simulink model "three_ringnetwork_with_control"  (R2016a)
settings: Solver=VariableStepAuto  StartTime=0.0  StopTime=0.2  RelTol=1e-3
undefined symbols (not defined in the file): vc0d
libraries: simulink x18, powerlib_meascontrol x3
(part 1 of 3)
settings Model: Creator=r-manohar  LastModifiedBy=r-manohar

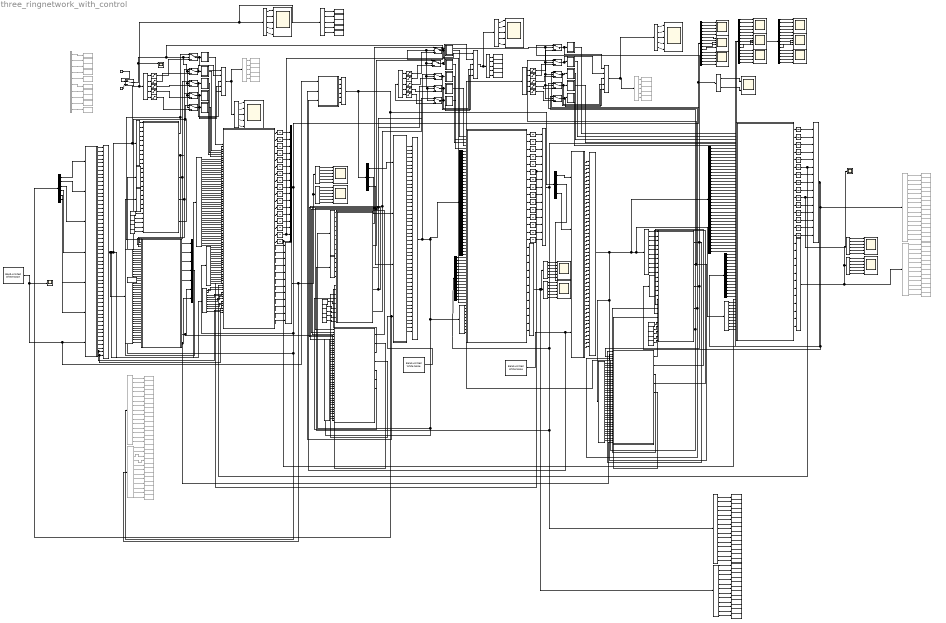
== system three_ringnetwork_with_control ==
  note: ab
  note: bc
  note: ca
  " Switch" : ManualSwitch
  Band-Limited White Noise : simulink/Sources/Band-Limited White Noise  Cov=[0.07]  Ts=0.01  seed=[234321]
  Band-Limited White Noise1 : simulink/Sources/Band-Limited White Noise  Cov=[0.07]  Ts=0.01  seed=[23341]
  Band-Limited White Noise2 : simulink/Sources/Band-Limited White Noise  Cov=[0.07]  Ts=0.01  seed=[2314441]
  Bus Creator1 : BusCreator  Inputs=17
  Bus Creator10 : BusCreator  Inputs=7
  Bus Creator11 : BusCreator  Inputs=6
  Bus Creator12 : BusCreator  Inputs=5
  Bus Creator13 : BusCreator  Inputs=5
  Bus Creator14 : BusCreator  Inputs=5
  Bus Creator2 : BusCreator  Inputs=56
  Bus Creator3 : BusCreator  Inputs=15
  Bus Creator4 : BusCreator  Inputs=12
  Bus Creator5 : BusCreator  Inputs=15
  Bus Creator6 : BusCreator  Inputs=12
  Bus Creator7 : BusCreator  Inputs=12
  Bus Creator8 : BusCreator  Inputs=50
  Bus Creator9 : BusCreator  Inputs=50
  Bus Selector1 : BusSelector  OutputSignals=E0,E1,E2,E3,E4,R1t0,R1t1,R1t2,R1t3,R1t4,R2t0,R2t1,R2t2,R2t3,R2t4,C0,C1,C2,C3,C4,L0,L1,L2,L3,L4,Lt0,Lt1,Lt2,Lt3,Lt4,il0d,il1d,il2d,il3d,il4d
  Bus Selector10 : BusSelector  OutputSignals=U0,U1,U2,U3,U4
  Bus Selector11 : BusSelector  OutputSignals=H,H0,H1,H2,H3,H4
  Bus Selector12 : BusSelector  OutputSignals=He0,He1,He2,He3,He4,He
  Bus Selector13 : BusSelector  OutputSignals=H,H0,H1,H2,H3,H4
  Bus Selector14 : BusSelector  OutputSignals=signal1,signal2,signal3,signal4,signal5,signal6,signal7,signal8,signal9,signal10,signal11,signal12,signal13,signal14,signal15,signal16,signal17
  Bus Selector{15..16,22..23,26,31,43..44} (8 alike) : BusSelector  OutputSignals=signal1,signal2,signal3,signal4,signal5
  Bus Selector17 : BusSelector  OutputSignals=He0,He1,He2,He3,He4,He
  Bus Selector18 : BusSelector  Commented=on  OutputSignals=signal1,signal2,signal3,signal4,signal5
  Bus Selector19 : BusSelector  OutputSignals=H,H0,H1,H2,H3,H4
  Bus Selector2 : BusSelector  OutputSignals=E0,E1,E2,E3,E4,R1t0,R1t1,R1t2,R1t3,R1t4,R2t0,R2t1,R2t2,R2t3,R2t4,C0,C1,C2,C3,C4,L0,L1,L2,L3,L4,Lt0,Lt1,Lt2,Lt3,Lt4,il0d,il1d,il2d,il3d,il4d,Rab,Lab,Rac,Lac
  Bus Selector20 : BusSelector  OutputSignals=vc0ss,vc1ss,vc2ss,vc3ss,vc4ss,ilt0ss,ilt1ss,ilt2ss,ilt3ss,ilt4ss
  Bus Selector21 : BusSelector  OutputSignals=E0,E1,E2,E3,E4,il0d,il1d,il2d,il3d,il4d
  Bus Selector24 : BusSelector  OutputSignals=R1t0,R1t1,R1t2,R1t3,R1t4,R2t0,R2t1,R2t2,R2t3,R2t4,il0d,il1d,il2d,il3d,il4d,C0,C1,C2,C3,C4,Lt0,Lt1,Lt2,Lt3,Lt4,vc0ss,vc1ss,vc2ss,vc3ss,vc4ss,ilt0ss,ilt1ss,ilt2ss,ilt3ss,ilt4ss,Lab,Lac,Rab,Rac,iabss,iacss
  Bus Selector25 : BusSelector  OutputSignals=E0,E1,E2,E3,E4,il0d,il1d,il2d,il3d,il4d
  Bus Selector{3,6..7,27,32,47} (6 alike) : BusSelector  OutputSignals=signal1,signal2,signal3,signal4,signal5,signal6,signal7,signal8,signal9,signal10,signal11,signal12,signal13,signal14,signal15
  Bus Selector28 : BusSelector  OutputSignals=R1t0,R1t1,R1t2,R1t3,R1t4,R2t0,R2t1,R2t2,R2t3,R2t4,il0d,il1d,il2d,il3d,il4d,C0,C1,C2,C3,C4,Lt0,Lt1,Lt2,Lt3,Lt4,vc0ss,vc1ss,vc2ss,vc3ss,vc4ss,ilt0ss,ilt1ss,ilt2ss,ilt3ss,ilt4ss
  Bus Selector29 : BusSelector  OutputSignals=R1t0,R1t1,R1t2,R1t3,R1t4,R2t0,R2t1,R2t2,R2t3,R2t4,il0d,il1d,il2d,il3d,il4d,C0,C1,C2,C3,C4,Lt0,Lt1,Lt2,Lt3,Lt4,vc0ss,vc1ss,vc2ss,vc3ss,vc4ss,ilt0ss,ilt1ss,ilt2ss,ilt3ss,ilt4ss
  Bus Selector30 : BusSelector  OutputSignals=E0,E1,E2,E3,E4,il0d,il1d,il2d,il3d,il4d
  Bus Selector33 : BusSelector  OutputSignals=Eb0,Rab,Ea0
  Bus Selector34 : BusSelector  OutputSignals=Ec0,Rac,Ea1
  Bus Selector35 : BusSelector  OutputSignals=Rab,Rac,Ea0,Ea1,Eb0,Ec0
  Bus Selector36 : BusSelector  OutputSignals=U0,U1,U2,U3,U4
  Bus Selector37 : BusSelector  OutputSignals=U0,U1,U2,U3,U4
  Bus Selector38 : BusSelector  Commented=on  OutputSignals=signal1,signal2,signal3,signal4,signal5,signal6,signal7,signal8,signal9,signal10,signal11,signal12,signal13,signal14,signal15
  Bus Selector39 : BusSelector  OutputSignals=signal16,signal17
  Bus Selector4 : BusSelector  OutputSignals=vc0ss,vc1ss,vc2ss,vc3ss,vc4ss,ilt0ss,ilt1ss,ilt2ss,ilt3ss,ilt4ss
  Bus Selector40 : BusSelector  Commented=on  OutputSignals=He0,He1,He2,He3,He4,He,H,H0,H1,H2,H3,H4
  Bus Selector41 : BusSelector  Commented=on  OutputSignals=E0,E1,E2,E3,E4,R2t0,R2t1,R2t2,R2t3,R2t4
  Bus Selector42 : BusSelector  OutputSignals=E0,E1,E2,E3,E4
  Bus Selector45 : BusSelector  OutputSignals=E0,E1,E2,E3,E4
  Bus Selector46 : BusSelector  Commented=on  OutputSignals=signal1,signal2,signal3,signal4,signal5
  Bus Selector48 : BusSelector  OutputSignals=He0,He1,He2,He3,He4,He,H,H0,H1,H2,H3,H4
  Bus Selector49 : BusSelector  Commented=on  OutputSignals=signal1,signal2,signal3,signal4,signal5,signal6,signal7,signal8,signal9,signal10,signal11,signal12,signal13,signal14,signal15
  Bus Selector5 : BusSelector  OutputSignals=E0,E1,E2,E3,E4,R1t0,R1t1,R1t2,R1t3,R1t4,R2t0,R2t1,R2t2,R2t3,R2t4,C0,C1,C2,C3,C4,L0,L1,L2,L3,L4,Lt0,Lt1,Lt2,Lt3,Lt4,il0d,il1d,il2d,il3d,il4d
  Bus Selector50 : BusSelector  Commented=on  OutputSignals=He0,He1,He2,He3,He4,He,H,H0,H1,H2,H3,H4
  Bus Selector8 : BusSelector  OutputSignals=vc0ss,vc1ss,vc2ss,vc3ss,vc4ss,ilt0ss,ilt1ss,ilt2ss,ilt3ss,ilt4ss
  Bus Selector9 : BusSelector  OutputSignals=He0,He1,He2,He3,He4,He
  Init : MATLAB Function  TreatAsAtomicUnit=on
  Init1 : MATLAB Function  TreatAsAtomicUnit=on
  Init2 : MATLAB Function  TreatAsAtomicUnit=on
  MATLAB Function : MATLAB Function  TreatAsAtomicUnit=on
  PWM0 : Subsystem
  PWM1 : Subsystem
  PWM10 : Subsystem
  PWM11 : Subsystem
  PWM12 : Subsystem
  PWM13 : Subsystem
  PWM14 : Subsystem
  PWM2 : Subsystem
  PWM3 : Subsystem
  PWM4 : Subsystem
  PWM5 : Subsystem
  PWM6 : Subsystem
  PWM7 : Subsystem
  PWM8 : Subsystem
  PWM9 : Subsystem
  Ralpha : Constant  Value=20
  Ralpha1 : Constant  Value=20
  Ralpha2 : Constant  Value=20
  Rbeta : Constant  Value=20
  Rbeta1 : Constant  Value=20
  Rbeta2 : Constant  Value=20
  Rdelta : Constant  Value=20
  Rdelta1 : Constant  Value=20
  Rdelta2 : Constant  Value=20
  Reta : Constant  Value=20
  Reta1 : Constant  Value=20
  Reta2 : Constant  Value=20
  Rgamma : Constant  Value=20
  Rgamma1 : Constant  Value=20
  Rgamma2 : Constant  Value=20
  Saturation{,1..14} (15 alike) : Saturate  UpperLimit=1  LowerLimit=0
  Scope : Scope
  Scope1 : Scope  NumInputPorts=2
  Scope4 : Scope  NumInputPorts=2
  Switch{,1..14} (15 alike) : Switch  Criteria=u2 > Threshold  Threshold=0.5
  cont : Subsystem
  cont1 : Subsystem
  cont2 : Subsystem
  controll : Constant
  h : Scope  NumInputPorts=6
  h1 : Scope  NumInputPorts=6
  h2 : Scope  NumInputPorts=6
  he : Scope  NumInputPorts=6
  he0_file1 : ToFile  Commented=on  Filename=E0.mat  MatrixName=E0_tr
  he0_file10 : ToFile  Filename=E0.mat  MatrixName=E0_tr
  he0_file11 : ToFile  Filename=h4.mat  MatrixName=h4_tr
  he0_file12 : ToFile  Commented=on  Filename=h4.mat  MatrixName=h4_tr
  he0_file13 : ToFile  Commented=on  Filename=he0.mat  MatrixName=he0_tr
  he0_file14 : ToFile  Commented=on  Filename=h3.mat  MatrixName=h3_tr
  he0_file15 : ToFile  Commented=on  Filename=h0.mat  MatrixName=h0_tr
  he0_file2 : ToFile  Commented=on  Filename=R2t0.mat  MatrixName=R2t0_tr
  he0_file3 : ToFile  Commented=on  Filename=he0.mat  MatrixName=he0_tr
  he0_file4 : ToFile  Commented=on  Filename=h3.mat  MatrixName=h3_tr
  he0_file5 : ToFile  Commented=on  Filename=h0.mat  MatrixName=h0_tr
  he0_file6 : ToFile  Commented=on  Filename=h4.mat  MatrixName=h4_tr
  he0_file7 : ToFile  Filename=he0.mat  MatrixName=he0_tr
  he0_file8 : ToFile  Filename=h3.mat  MatrixName=h3_tr
  he0_file9 : ToFile  Filename=h0.mat  MatrixName=h0_tr
  he1 : Scope  NumInputPorts=6
  he1_file1 : ToFile  Filename=he1.mat  MatrixName=he1_tr
  he1_file10 : ToFile  Commented=on  Filename=E2.mat  MatrixName=E2_tr
  he1_file11 : ToFile  Commented=on  Filename=E3.mat  MatrixName=E3_tr
  he1_file12 : ToFile  Commented=on  Filename=E4.mat  MatrixName=E4_tr
  he1_file13 : ToFile  Commented=on  Filename=R2t2.mat  MatrixName=R2t2_tr
  he1_file14 : ToFile  Commented=on  Filename=R2t3.mat  MatrixName=R2t3_tr
  he1_file15 : ToFile  Commented=on  Filename=R2t4.mat  MatrixName=R2t4_tr
  he1_file16 : ToFile  Commented=on  Filename=R2t1.mat  MatrixName=R2t1_tr
  he1_file17 : ToFile  Commented=on  Filename=h2.mat  MatrixName=h2_tr
  he1_file2 : ToFile  Filename=h1.mat  MatrixName=h1_tr
  he1_file24 : ToFile  Filename=E2.mat  MatrixName=E2_tr
  he1_file25 : ToFile  Filename=E3.mat  MatrixName=E3_tr
  he1_file26 : ToFile  Filename=E4.mat  MatrixName=E4_tr
  he1_file27 : ToFile  Filename=E1.mat  MatrixName=E1_tr
  he1_file3 : ToFile  Commented=on  Filename=he1.mat  MatrixName=he1_tr
  he1_file4 : ToFile  Commented=on  Filename=h1.mat  MatrixName=h1_tr
  he1_file5 : ToFile  Commented=on  Filename=h2.mat  MatrixName=h2_tr
  he1_file6 : ToFile  Filename=h2.mat  MatrixName=h2_tr
  he1_file7 : ToFile  Commented=on  Filename=he1.mat  MatrixName=he1_tr
  he1_file8 : ToFile  Commented=on  Filename=h1.mat  MatrixName=h1_tr
  he1_file9 : ToFile  Commented=on  Filename=E1.mat  MatrixName=E1_tr
  he2 : Scope  NumInputPorts=6
  he2_file1 : ToFile  Commented=on  Filename=he2.mat  MatrixName=he2_tr
  he2_file2 : ToFile  Filename=he2.mat  MatrixName=he2_tr
  he2_file3 : ToFile  Commented=on  Filename=he2.mat  MatrixName=he2_tr
  he3 : Scope  NumInputPorts=2
  he_file1 : ToFile  Filename=he.mat  MatrixName=he_tr
  he_file10 : ToFile  Commented=on  Filename=he.mat  MatrixName=he_tr
  he_file11 : ToFile  Commented=on  Filename=h.mat  MatrixName=h_tr
  he_file12 : ToFile  Commented=on  Filename=he3.mat  MatrixName=he3_tr
  he_file13 : ToFile  Commented=on  Filename=he4.mat  MatrixName=he4_tr
  he_file2 : ToFile  Filename=h.mat  MatrixName=h_tr
  he_file3 : ToFile  Filename=he3.mat  MatrixName=he3_tr
  he_file4 : ToFile  Commented=on  Filename=he.mat  MatrixName=he_tr
  he_file5 : ToFile  Filename=iltd  MatrixName=iltd_tr
  he_file6 : ToFile  Commented=on  Filename=h.mat  MatrixName=h_tr
  he_file7 : ToFile  Commented=on  Filename=he3.mat  MatrixName=he3_tr
  he_file8 : ToFile  Commented=on  Filename=he4.mat  MatrixName=he4_tr
  he_file9 : ToFile  Filename=he4.mat  MatrixName=he4_tr
  il : Scope  NumInputPorts=5
  il{0..14} (15 alike) : Integrator
  il0_file1 : ToFile  Commented=on  Filename=duty_0.mat  MatrixName=duty_0_tr
  il0_file10 : ToFile  Filename=vc3.mat  MatrixName=vc3_tr
  il0_file11 : ToFile  Filename=vc4.mat  MatrixName=vc4_tr
  il0_file12 : ToFile  Commented=on  Filename=vc3.mat  MatrixName=vc3_tr
  il0_file13 : ToFile  Commented=on  Filename=vc4.mat  MatrixName=vc4_tr
  il0_file14 : ToFile  Commented=on  Filename=il0.mat  MatrixName=il0_tr
  il0_file15 : ToFile  Commented=on  Filename=vc0.mat  MatrixName=vc0_tr
  il0_file2 : ToFile  Commented=on  Filename=duty_0.mat  MatrixName=duty_0_tr
  il0_file3 : ToFile  Filename=il0.mat  MatrixName=il0_tr
  il0_file4 : ToFile  Filename=duty_0.mat  MatrixName=duty_0_tr
  il0_file5 : ToFile  Commented=on  Filename=il0.mat  MatrixName=il0_tr
  il0_file6 : ToFile  Commented=on  Filename=vc0.mat  MatrixName=vc0_tr
  il0_file7 : ToFile  Commented=on  Filename=vc3.mat  MatrixName=vc3_tr
  il0_file8 : ToFile  Commented=on  Filename=vc4.mat  MatrixName=vc4_tr
  il0_file9 : ToFile  Filename=vc0.mat  MatrixName=vc0_tr
  il15 : Scope  NumInputPorts=5
  il16 : Scope  NumInputPorts=5
  il1_file1 : ToFile  Filename=duty_1.mat  MatrixName=duty_1_tr
  il1_file2 : ToFile  Commented=on  Filename=il1.mat  MatrixName=il1_tr
  il1_file3 : ToFile  Commented=on  Filename=duty_1.mat  MatrixName=duty_1_tr
  il1_file4 : ToFile  Commented=on  Filename=duty_1.mat  MatrixName=duty_1_tr
  il1_file5 : ToFile  Filename=il1.mat  MatrixName=il1_tr
  il1_file6 : ToFile  Commented=on  Filename=il1.mat  MatrixName=il1_tr
  il2_file1 : ToFile  Commented=on  Filename=duty_2.mat  MatrixName=duty_2_tr
  il2_file10 : ToFile  Commented=on  Filename=duty_2.mat  MatrixName=duty_2_tr
  il2_file11 : ToFile  Commented=on  Filename=duty_4.mat  MatrixName=duty_4_tr
  il2_file12 : ToFile  Commented=on  Filename=duty_3.mat  MatrixName=duty_3_tr
  il2_file13 : ToFile  Filename=il2.mat  MatrixName=il2_tr
  il2_file14 : ToFile  Filename=il3.mat  MatrixName=il3_tr
  il2_file15 : ToFile  Filename=il4.mat  MatrixName=il4_tr
  il2_file16 : ToFile  Commented=on  Filename=il2.mat  MatrixName=il2_tr
  il2_file17 : ToFile  Commented=on  Filename=il3.mat  MatrixName=il3_tr
  il2_file18 : ToFile  Commented=on  Filename=il4.mat  MatrixName=il4_tr
  il2_file2 : ToFile  Commented=on  Filename=duty_4.mat  MatrixName=duty_4_tr
  il2_file3 : ToFile  Filename=duty_2.mat  MatrixName=duty_2_tr
  il2_file4 : ToFile  Filename=duty_4.mat  MatrixName=duty_4_tr
  il2_file5 : ToFile  Filename=duty_3.mat  MatrixName=duty_3_tr
  il2_file6 : ToFile  Commented=on  Filename=il2.mat  MatrixName=il2_tr
  il2_file7 : ToFile  Commented=on  Filename=il3.mat  MatrixName=il3_tr
  il2_file8 : ToFile  Commented=on  Filename=il4.mat  MatrixName=il4_tr
  il2_file9 : ToFile  Commented=on  Filename=duty_3.mat  MatrixName=duty_3_tr
  ilt{,5,7,21..24} (7 alike) : Scope  NumInputPorts=5
  ilt{0..4,6,8..20} (19 alike) : Integrator
  ilt0_file1 : ToFile  Filename=ilt0.mat  MatrixName=ilt0_tr
  ilt0_file2 : ToFile  Filename=ilt4.mat  MatrixName=ilt4_tr
  ilt0_file3 : ToFile  Commented=on  Filename=ilt0.mat  MatrixName=ilt0_tr
  ilt0_file4 : ToFile  Commented=on  Filename=ilt4.mat  MatrixName=ilt4_tr
  ilt0_file5 : ToFile  Commented=on  Filename=ilt3.mat  MatrixName=ilt3_tr
  ilt0_file6 : ToFile  Filename=ilt3.mat  MatrixName=ilt3_tr
  ilt0_file7 : ToFile  Commented=on  Filename=ilt0.mat  MatrixName=ilt0_tr
  ilt0_file8 : ToFile  Commented=on  Filename=ilt4.mat  MatrixName=ilt4_tr
  ilt0_file9 : ToFile  Commented=on  Filename=ilt3.mat  MatrixName=ilt3_tr
  ilt1_file1 : ToFile  Commented=on  Filename=ilt1.mat  MatrixName=ilt1_tr
  ilt1_file2 : ToFile  Filename=ilt1.mat  MatrixName=ilt1_tr
  ilt1_file3 : ToFile  Commented=on  Filename=ilt1.mat  MatrixName=ilt1_tr
  ilt2_file1 : ToFile  Commented=on  Filename=ilt2.mat  MatrixName=ilt2_tr
  ilt2_file2 : ToFile  Filename=ilt2.mat  MatrixName=ilt2_tr
  ilt2_file3 : ToFile  Commented=on  Filename=ilt2.mat  MatrixName=ilt2_tr
  "nocontrol " : Constant  Value=0
  utt : Subsystem
  utt1 : Subsystem
  utt2 : Subsystem
  vc : Scope  NumInputPorts=6
  vc{0..5,7..9,11..14} (13 alike) : Integrator
  vc10 : Scope  NumInputPorts=6
  vc1_file1 : ToFile  Commented=on  Filename=vc1.mat  MatrixName=vc1_tr
  vc1_file2 : ToFile  Filename=vc1.mat  MatrixName=vc1_tr
  vc1_file3 : ToFile  Commented=on  Filename=vc1.mat  MatrixName=vc1_tr
  vc2_file1 : ToFile  Commented=on  Filename=vc2.mat  MatrixName=vc2_tr
  vc2_file2 : ToFile  Filename=vc2.mat  MatrixName=vc2_tr
  vc2_file3 : ToFile  Commented=on  Filename=vc2.mat  MatrixName=vc2_tr
  vc6 : Scope  NumInputPorts=6
  whole_sys : MATLAB Function  TreatAsAtomicUnit=on
  whole_sys1 : MATLAB Function  TreatAsAtomicUnit=on
  whole_sys2 : MATLAB Function  TreatAsAtomicUnit=on
  wires:
  Bus Selector10/1 -> Saturation/1  "<U0>"
  Bus Selector10/2 -> Saturation1/1  "<U1>"
  Bus Selector10/3 -> Saturation2/1  "<U2>"
  controll/1 -> " Switch"/1
  Bus Creator4/1 -> Bus Selector50/1, Bus Selector12/1, Bus Selector13/1
  Bus Selector12/1 -> he/1  "<He0>"
  Bus Selector12/2 -> he/2  "<He1>"
  Bus Selector12/3 -> he/3  "<He2>"
  Bus Selector3/1 -> il/1  "<signal1>"
  Bus Selector3/3 -> il/3  "<signal3>"
  Bus Selector3/4 -> il/4  "<signal4>"
  Bus Selector3/5 -> il/5  "<signal5>"
  Bus Selector3/6 -> vc/1  "<signal6>"
  Bus Selector3/8 -> vc/3  "<signal8>"
  Bus Selector3/9 -> vc/4  "<signal9>"
  Bus Selector3/10 -> vc/5  "<signal10>"
  Bus Selector3/12 -> ilt/2  "<signal12>"
  Bus Selector3/11 -> ilt/1  "<signal11>"
  Bus Selector3/13 -> ilt/3  "<signal13>"
  Bus Selector3/14 -> ilt/4  "<signal14>"
  Bus Selector3/15 -> ilt/5  "<signal15>"
  Bus Selector12/4 -> he/4  "<He3>"
  Bus Selector12/5 -> he/5  "<He4>"
  Bus Selector12/6 -> he/6  "<He>"
  Bus Selector13/1 -> h/1  "<H>"
  Bus Selector13/2 -> h/2  "<H0>"
  Bus Selector13/3 -> h/3  "<H1>"
  Bus Selector13/4 -> h/4  "<H2>"
  Bus Selector13/5 -> h/5  "<H3>"
  Bus Selector13/6 -> h/6  "<H4>"
  ? -> ?
  Bus Selector4/1 -> whole_sys/64(vc0d)  "<vc0ss>"
  Bus Selector4/2 -> whole_sys/65(vc1d)  "<vc1ss>"
  Bus Selector4/3 -> whole_sys/66(vc2d)  "<vc2ss>"
  Bus Selector4/4 -> whole_sys/67(vc3d)  "<vc3ss>"
  Bus Selector4/5 -> whole_sys/68(vc4d)  "<vc4ss>"
  Bus Selector4/6 -> whole_sys/69(ilt0d)  "<ilt0ss>"
  Bus Selector4/7 -> whole_sys/70(ilt1d)  "<ilt1ss>"
  Bus Selector4/8 -> whole_sys/71(ilt2d)  "<ilt2ss>"
  Bus Selector4/9 -> whole_sys/72(ilt3d)  "<ilt3ss>"
  Bus Selector4/10 -> whole_sys/73(ilt4d)  "<ilt4ss>"
  Bus Selector10/4 -> Saturation3/1  "<U3>"
  PWM0/1(P) -> whole_sys/1(u0)
  PWM1/1(P) -> whole_sys/2(u1)
  PWM2/1(P) -> whole_sys/3(u2)
  PWM3/1(P) -> whole_sys/4(u3)
  PWM4/1(P) -> whole_sys/5(u4)
  Bus Selector10/5 -> Saturation4/1  "<U4>"
  Bus Selector3/2 -> il/2  "<signal2>"
  Bus Selector3/7 -> vc/2  "<signal7>"
  whole_sys1/1(il0dot) -> il5/1
  whole_sys1/9(vc3dot) -> vc9/1
  whole_sys1/2(il1dot) -> il6/1
  whole_sys1/3(il2dot) -> il7/1
  whole_sys1/4(il3dot) -> il8/1
  whole_sys1/5(il4dot) -> il9/1
  whole_sys1/6(vc0dot) -> vc5/1
  whole_sys1/15(ilt4dot) -> ilt14/1
  whole_sys1/14(ilt3dot) -> ilt13/1
  whole_sys1/13(ilt2dot) -> ilt12/1
  whole_sys1/12(ilt1dot) -> ilt11/1
  whole_sys1/11(ilt0dot) -> ilt10/1
  whole_sys1/10(vc4dot) -> ilt9/1
  whole_sys1/7(vc1dot) -> vc7/1
  whole_sys1/8(vc2dot) -> vc8/1
  whole_sys2/1(il0dot) -> il10/1
  whole_sys2/2(il1dot) -> il11/1
  whole_sys2/3(il2dot) -> il12/1
  whole_sys2/4(il3dot) -> il13/1
  whole_sys2/5(il4dot) -> il14/1
  whole_sys2/6(vc0dot) -> vc11/1
  whole_sys2/7(vc1dot) -> vc12/1
  whole_sys2/8(vc2dot) -> vc13/1
  whole_sys2/9(vc3dot) -> vc14/1
  whole_sys2/10(vc4dot) -> ilt15/1
  whole_sys2/11(ilt0dot) -> ilt16/1
  whole_sys2/12(ilt1dot) -> ilt17/1
  whole_sys2/13(ilt2dot) -> ilt18/1
  whole_sys2/14(ilt3dot) -> ilt19/1
  Bus Selector14/1 -> whole_sys/45(il0)  "<signal1>"
  Bus Selector14/2 -> whole_sys/46(il1)  "<signal2>"
  Bus Selector14/3 -> whole_sys/47(il2)  "<signal3>"
  Bus Selector14/4 -> whole_sys/48(il3)  "<signal4>"
  Bus Selector14/5 -> whole_sys/49(il4)  "<signal5>"
  Bus Selector14/6 -> whole_sys/50(vc0)  "<signal6>"
  Bus Selector14/7 -> whole_sys/51(vc1)  "<signal7>"
  Bus Selector14/8 -> whole_sys/52(vc2)  "<signal8>"
  Bus Selector14/9 -> whole_sys/53(vc3)  "<signal9>"
  Bus Selector14/10 -> whole_sys/54(vc4)  "<signal10>"
  Bus Selector14/11 -> whole_sys/55(ilt0)  "<signal11>"
  Bus Selector14/12 -> whole_sys/56(ilt1)  "<signal12>"
  Bus Selector14/13 -> whole_sys/57(ilt2)  "<signal13>"
  Bus Selector14/14 -> whole_sys/58(ilt3)  "<signal14>"
  Bus Selector14/15 -> whole_sys/59(ilt4)  "<signal15>"
  Bus Selector14/16 -> whole_sys/60(iab)  "<signal16>"
  Bus Selector14/17 -> whole_sys/61(iac)  "<signal17>"
  Bus Selector2/1 -> whole_sys/6(E0)  "<E0>"
  Bus Selector2/2 -> whole_sys/7(E1)  "<E1>"
  Bus Selector2/3 -> whole_sys/8(E2)  "<E2>"
  Bus Selector2/4 -> whole_sys/9(E3)  "<E3>"
  Bus Selector2/5 -> whole_sys/10(E4)  "<E4>"
  Bus Selector2/6 -> whole_sys/11(R1t0)  "<R1t0>"
  Bus Selector2/7 -> whole_sys/12(R1t1)  "<R1t1>"
  Bus Selector2/8 -> whole_sys/13(R1t2)  "<R1t2>"
  Bus Selector2/9 -> whole_sys/14(R1t3)  "<R1t3>"
  Bus Selector2/10 -> whole_sys/15(R1t4)  "<R1t4>"
  Bus Selector2/11 -> whole_sys/16(R2t0)  "<R2t0>"
  Bus Selector2/12 -> whole_sys/17(R2t1)  "<R2t1>"
  Bus Selector2/13 -> whole_sys/18(R2t2)  "<R2t2>"
  Bus Selector2/14 -> whole_sys/19(R2t3)  "<R2t3>"
  Bus Selector2/15 -> whole_sys/20(R2t4)  "<R2t4>"
  Bus Selector2/16 -> whole_sys/21(C0)  "<C0>"
  Bus Selector2/17 -> whole_sys/22(C1)  "<C1>"
  Bus Selector2/18 -> whole_sys/23(C2)  "<C2>"
  Bus Selector2/19 -> whole_sys/24(C3)  "<C3>"
  Bus Selector2/20 -> whole_sys/25(C4)  "<C4>"
  Bus Selector2/21 -> whole_sys/26(L0)  "<L0>"
  Bus Selector2/22 -> whole_sys/27(L1)  "<L1>"
  Bus Selector2/23 -> whole_sys/28(L2)  "<L2>"
  Bus Selector2/24 -> whole_sys/29(L3)  "<L3>"
  Bus Selector2/25 -> whole_sys/30(L4)  "<L4>"
  Bus Selector2/26 -> whole_sys/31(Lt0)  "<Lt0>"
  Bus Selector2/27 -> whole_sys/32(Lt1)  "<Lt1>"
  Bus Selector2/28 -> whole_sys/33(Lt2)  "<Lt2>"
  Bus Selector2/29 -> whole_sys/34(Lt3)  "<Lt3>"
  Bus Selector2/30 -> whole_sys/35(Lt4)  "<Lt4>"
  Bus Selector2/31 -> whole_sys/36(il0d)  "<il0d>"
  Bus Selector2/32 -> whole_sys/37(il1d)  "<il1d>"
  Bus Selector2/33 -> whole_sys/38(il2d)  "<il2d>"
  Bus Selector2/34 -> whole_sys/39(il3d)  "<il3d>"
  Bus Selector2/35 -> whole_sys/40(il4d)  "<il4d>"
  Bus Selector2/36 -> whole_sys/41(Rab)  "<Rab>"
  Bus Selector2/37 -> whole_sys/42(Lab)  "<Lab>"
  Bus Selector2/38 -> whole_sys/43(Rac)  "<Rac>"
  Bus Selector2/39 -> whole_sys/44(Lac)  "<Lac>"
  il5/1 -> Bus Creator3/1
  il6/1 -> Bus Creator3/2
  il7/1 -> Bus Creator3/3
  il8/1 -> Bus Creator3/4
  il9/1 -> Bus Creator3/5
  vc7/1 -> Bus Creator3/7
  vc8/1 -> Bus Creator3/8
  vc9/1 -> Bus Creator3/9
  ilt9/1 -> Bus Creator3/10
  ilt10/1 -> Bus Creator3/11
  ilt11/1 -> Bus Creator3/12
  ilt12/1 -> Bus Creator3/13
  ilt13/1 -> Bus Creator3/14
  ilt14/1 -> Bus Creator3/15
  whole_sys2/15(ilt4dot) -> ilt20/1
  il10/1 -> Bus Creator5/1
  il11/1 -> Bus Creator5/2
  il12/1 -> Bus Creator5/3
  il13/1 -> Bus Creator5/4
  il14/1 -> Bus Creator5/5
  vc11/1 -> whole_sys/63(vc0c), Bus Creator5/6
  vc12/1 -> Bus Creator5/7
  vc13/1 -> Bus Creator5/8
  vc14/1 -> Bus Creator5/9
  ilt15/1 -> Scope/1, Bus Creator5/10
  ilt16/1 -> Bus Creator5/11
  ilt17/1 -> Bus Creator5/12
  ilt18/1 -> Bus Creator5/13
  ilt19/1 -> Bus Creator5/14
  ilt20/1 -> Bus Creator5/15
  Bus Selector7/1 -> whole_sys2/41(il0)  "<signal1>"
  Bus Selector7/2 -> whole_sys2/42(il1)  "<signal2>"
  Bus Selector7/3 -> whole_sys2/43(il2)  "<signal3>"
  Bus Selector7/4 -> whole_sys2/44(il3)  "<signal4>"
  Bus Selector7/5 -> whole_sys2/45(il4)  "<signal5>"
  Bus Selector7/6 -> whole_sys2/46(vc0)  "<signal6>"
  Bus Selector7/7 -> whole_sys2/47(vc1)  "<signal7>"
  Bus Selector7/8 -> whole_sys2/48(vc2)  "<signal8>"
  Bus Selector7/9 -> whole_sys2/49(vc3)  "<signal9>"
  Bus Selector7/10 -> whole_sys2/50(vc4)  "<signal10>"
  Bus Selector7/11 -> whole_sys2/51(ilt0)  "<signal11>"
  Bus Selector7/12 -> whole_sys2/52(ilt1)  "<signal12>"
  Bus Selector7/13 -> whole_sys2/53(ilt2)  "<signal13>"
  Bus Selector7/14 -> whole_sys2/54(ilt3)  "<signal14>"
  Bus Selector7/15 -> whole_sys2/55(ilt4)  "<signal15>"
  Bus Selector20/1 -> whole_sys2/57(vc0d)  "<vc0ss>"
  Bus Selector20/2 -> whole_sys2/58(vc1d)  "<vc1ss>"
  Bus Selector20/3 -> whole_sys2/59(vc2d)  "<vc2ss>"
  Bus Selector20/4 -> whole_sys2/60(vc3d)  "<vc3ss>"
  Bus Selector20/5 -> whole_sys2/61(vc4d)  "<vc4ss>"
  Bus Selector20/6 -> whole_sys2/62(ilt0d)  "<ilt0ss>"
  Bus Selector20/7 -> whole_sys2/63(ilt1d)  "<ilt1ss>"
  Bus Selector20/8 -> whole_sys2/64(ilt2d)  "<ilt2ss>"
  Bus Selector20/9 -> whole_sys2/65(ilt3d)  "<ilt3ss>"
  Bus Selector20/10 -> whole_sys2/66(ilt4d)  "<ilt4ss>"
  Bus Selector5/1 -> whole_sys2/6(E0)  "<E0>"
  Bus Selector5/2 -> whole_sys2/7(E1)  "<E1>"
  Bus Selector5/3 -> whole_sys2/8(E2)  "<E2>"
  Bus Selector5/4 -> whole_sys2/9(E3)  "<E3>"
  Bus Selector5/5 -> whole_sys2/10(E4)  "<E4>"
  Bus Selector5/6 -> whole_sys2/11(R1t0)  "<R1t0>"
  Bus Selector5/7 -> whole_sys2/12(R1t1)  "<R1t1>"
  Bus Selector5/8 -> whole_sys2/13(R1t2)  "<R1t2>"
  Bus Selector5/9 -> whole_sys2/14(R1t3)  "<R1t3>"
  Bus Selector5/10 -> whole_sys2/15(R1t4)  "<R1t4>"
  Bus Selector5/11 -> whole_sys2/16(R2t0)  "<R2t0>"
  Bus Selector5/12 -> whole_sys2/17(R2t1)  "<R2t1>"
  Bus Selector5/13 -> whole_sys2/18(R2t2)  "<R2t2>"
  Bus Selector5/14 -> whole_sys2/19(R2t3)  "<R2t3>"
  Bus Selector5/15 -> whole_sys2/20(R2t4)  "<R2t4>"
  Bus Selector5/16 -> whole_sys2/21(C0)  "<C0>"
  Bus Selector5/17 -> whole_sys2/22(C1)  "<C1>"
  Bus Selector5/18 -> whole_sys2/23(C2)  "<C2>"
  Bus Selector5/19 -> whole_sys2/24(C3)  "<C3>"
  Bus Selector5/20 -> whole_sys2/25(C4)  "<C4>"
  Bus Selector5/21 -> whole_sys2/26(L0)  "<L0>"
  Bus Selector5/22 -> whole_sys2/27(L1)  "<L1>"
  Bus Selector5/23 -> whole_sys2/28(L2)  "<L2>"
  Bus Selector5/24 -> whole_sys2/29(L3)  "<L3>"
  Bus Selector5/25 -> whole_sys2/30(L4)  "<L4>"
  Bus Selector5/26 -> whole_sys2/31(Lt0)  "<Lt0>"
  Bus Selector5/27 -> whole_sys2/32(Lt1)  "<Lt1>"
  Bus Selector5/28 -> whole_sys2/33(Lt2)  "<Lt2>"
  Bus Selector5/29 -> whole_sys2/34(Lt3)  "<Lt3>"
  Bus Selector5/30 -> whole_sys2/35(Lt4)  "<Lt4>"
  Bus Selector5/31 -> whole_sys2/36(il0d)  "<il0d>"
  Bus Selector5/32 -> whole_sys2/37(il1d)  "<il1d>"
  Bus Selector5/33 -> whole_sys2/38(il2d)  "<il2d>"
  Bus Selector5/34 -> whole_sys2/39(il3d)  "<il3d>"
  Bus Selector5/35 -> whole_sys2/40(il4d)  "<il4d>"
  whole_sys/18(He0) -> Bus Creator4/1
  whole_sys/19(He1) -> Bus Creator4/2
  whole_sys/20(He2) -> Bus Creator4/3
  whole_sys/21(He3) -> Bus Creator4/4
  whole_sys/22(He4) -> Bus Creator4/5
  whole_sys/23(He) -> Bus Creator4/6
  whole_sys/24(H) -> Bus Creator4/7
  whole_sys/25(H0) -> Bus Creator4/8
  whole_sys/26(H1) -> Bus Creator4/9
  whole_sys/27(H2) -> Bus Creator4/10
  whole_sys/28(H3) -> Bus Creator4/11
  whole_sys/29(H4) -> Bus Creator4/12
  whole_sys1/16(He0) -> Bus Creator6/1
  whole_sys1/17(He1) -> Bus Creator6/2
  whole_sys1/18(He2) -> Bus Creator6/3
  whole_sys1/19(He3) -> Bus Creator6/4
  whole_sys1/20(He4) -> Bus Creator6/5
  whole_sys1/21(He) -> Bus Creator6/6
  whole_sys1/22(H) -> Bus Creator6/7
  whole_sys1/23(H0) -> Bus Creator6/8
  whole_sys1/24(H1) -> Bus Creator6/9
  whole_sys1/25(H2) -> Bus Creator6/10
  whole_sys1/26(H3) -> Bus Creator6/11
  whole_sys1/27(H4) -> Bus Creator6/12
  Bus Selector9/1 -> he1/1  "<He0>"
  Bus Selector9/2 -> he1/2  "<He1>"
  Bus Selector9/3 -> he1/3  "<He2>"
  Bus Selector9/4 -> he1/4  "<He3>"
  Bus Selector9/5 -> he1/5  "<He4>"
  Bus Selector9/6 -> he1/6  "<He>"
  Bus Selector11/1 -> h1/1  "<H>"
  Bus Selector11/2 -> h1/2  "<H0>"
  Bus Selector11/3 -> h1/3  "<H1>"
  Bus Selector11/4 -> h1/4  "<H2>"
  Bus Selector11/5 -> h1/5  "<H3>"
  Bus Selector11/6 -> h1/6  "<H4>"
  Bus Selector17/1 -> he2/1  "<He0>"
  Bus Selector17/2 -> he2/2  "<He1>"
  Bus Selector17/3 -> he2/3  "<He2>"
  ? -> ?
  Bus Selector17/4 -> he2/4  "<He3>"
  Bus Selector17/5 -> he2/5  "<He4>"
  Bus Selector17/6 -> he2/6  "<He>"
  Bus Selector19/1 -> h2/1  "<H>"
  Bus Selector19/2 -> h2/2  "<H0>"
  Bus Selector19/3 -> h2/3  "<H1>"
  Bus Selector19/4 -> h2/4  "<H2>"
  Bus Selector19/5 -> h2/5  "<H3>"
  Bus Selector19/6 -> h2/6  "<H4>"
  whole_sys2/16(He0) -> Bus Creator7/1
  whole_sys2/17(He1) -> Bus Creator7/2
  whole_sys2/18(He2) -> Bus Creator7/3
  whole_sys2/19(He3) -> Bus Creator7/4
  whole_sys2/20(He4) -> Bus Creator7/5
  whole_sys2/21(He) -> Bus Creator7/6
  whole_sys2/22(H) -> Bus Creator7/7
  whole_sys2/23(H0) -> Bus Creator7/8
  whole_sys2/24(H1) -> Bus Creator7/9
  whole_sys2/25(H2) -> Bus Creator7/10
  whole_sys2/26(H3) -> Bus Creator7/11
  whole_sys2/27(H4) -> Bus Creator7/12
  PWM5/1(P) -> whole_sys1/1(u0)
  PWM6/1(P) -> whole_sys1/2(u1)
  PWM7/1(P) -> whole_sys1/3(u2)
  PWM8/1(P) -> whole_sys1/4(u3)
  PWM10/1(P) -> whole_sys2/1(u0)
  PWM11/1(P) -> whole_sys2/2(u1)
  PWM12/1(P) -> whole_sys2/3(u2)
  PWM13/1(P) -> whole_sys2/4(u3)
  PWM14/1(P) -> whole_sys2/5(u4)
  Init1/1(E0) -> Bus Creator8/1
  Init1/2(E1) -> Bus Creator8/2
  Init1/3(E2) -> Bus Creator8/3
  Init1/4(E3) -> Bus Creator8/4
  Init1/5(E4) -> Bus Creator8/5
  Init1/6(U0) -> Bus Creator8/6
  Init1/7(U1) -> Bus Creator8/7
  Init1/8(U2) -> Bus Creator8/8
  Init1/9(U3) -> Bus Creator8/9
  Init1/10(U4) -> Bus Creator8/10
  Init1/11(R1t0) -> Bus Creator8/11
  Init1/12(R1t1) -> Bus Creator8/12
  Init1/13(R1t2) -> Bus Creator8/13
  Init1/14(R1t3) -> Bus Creator8/14
  Init1/15(R1t4) -> Bus Creator8/15
  Init1/16(R2t0) -> Bus Creator8/16
  Init1/17(R2t1) -> Bus Creator8/17
  Init1/18(R2t2) -> Bus Creator8/18
  Init1/19(R2t3) -> Bus Creator8/19
  Init1/20(R2t4) -> Bus Creator8/20
  Init1/21(C0) -> Bus Creator8/21
  Init1/22(C1) -> Bus Creator8/22
  Init1/23(C2) -> Bus Creator8/23
  Init1/24(C3) -> Bus Creator8/24
  Init1/25(C4) -> Bus Creator8/25
  Init1/26(L0) -> Bus Creator8/26
  Init1/27(L1) -> Bus Creator8/27
  Init1/28(L2) -> Bus Creator8/28
  Init1/29(L3) -> Bus Creator8/29
  Init1/30(L4) -> Bus Creator8/30
  Init1/31(Lt0) -> Bus Creator8/31
  Init1/32(Lt1) -> Bus Creator8/32
  Init1/33(Lt2) -> Bus Creator8/33
  Init1/34(Lt3) -> Bus Creator8/34
  Init1/35(Lt4) -> Bus Creator8/35
  Init1/36(il0d) -> Bus Creator8/36
  Init1/37(il1d) -> Bus Creator8/37
  Init1/38(il2d) -> Bus Creator8/38
  Init1/39(il3d) -> Bus Creator8/39
  Init1/40(il4d) -> Bus Creator8/40
  Init1/42(vc1ss) -> Bus Creator8/42
  Init1/43(vc2ss) -> Bus Creator8/43
  Init1/44(vc3ss) -> Bus Creator8/44
  Init1/45(vc4ss) -> Bus Creator8/45
  Init1/46(ilt0ss) -> Bus Creator8/46
  Init1/47(ilt1ss) -> Bus Creator8/47
  Init1/48(ilt2ss) -> Bus Creator8/48
  Init1/49(ilt3ss) -> Bus Creator8/49
  Init1/50(ilt4ss) -> Bus Creator8/50
  Init2/1(E0) -> Bus Creator9/1
  Init2/2(E1) -> Bus Creator9/2
  Init2/3(E2) -> Bus Creator9/3
  Init2/4(E3) -> Bus Creator9/4
  Init2/5(E4) -> Bus Creator9/5
  Init2/6(U0) -> Bus Creator9/6
  Init2/7(U1) -> Bus Creator9/7
  Init2/8(U2) -> Bus Creator9/8
  Init2/9(U3) -> Bus Creator9/9
  Init2/10(U4) -> Bus Creator9/10
  Init2/11(R1t0) -> Bus Creator9/11
  Init2/12(R1t1) -> Bus Creator9/12
  Init2/13(R1t2) -> Bus Creator9/13
  Init2/14(R1t3) -> Bus Creator9/14
  Init2/15(R1t4) -> Bus Creator9/15
  Init2/16(R2t0) -> Bus Creator9/16
  Init2/17(R2t1) -> Bus Creator9/17
  Init2/18(R2t2) -> Bus Creator9/18
  Init2/19(R2t3) -> Bus Creator9/19
  Init2/20(R2t4) -> Bus Creator9/20
  Init2/21(C0) -> Bus Creator9/21
  Init2/22(C1) -> Bus Creator9/22
  Init2/23(C2) -> Bus Creator9/23
  Init2/24(C3) -> Bus Creator9/24
  Init2/25(C4) -> Bus Creator9/25
  Init2/26(L0) -> Bus Creator9/26
  Init2/27(L1) -> Bus Creator9/27
  Init2/28(L2) -> Bus Creator9/28
  Init2/29(L3) -> Bus Creator9/29
  Init2/30(L4) -> Bus Creator9/30
  Init2/31(Lt0) -> Bus Creator9/31
  Init2/32(Lt1) -> Bus Creator9/32
  Init2/33(Lt2) -> Bus Creator9/33
  Init2/34(Lt3) -> Bus Creator9/34
  Init2/35(Lt4) -> Bus Creator9/35
  Init2/36(il0d) -> Bus Creator9/36
  Init2/37(il1d) -> Bus Creator9/37
  Init2/38(il2d) -> Bus Creator9/38
  Init2/39(il3d) -> Bus Creator9/39
  Init2/40(il4d) -> Bus Creator9/40
  Init2/41(vc0ss) -> Bus Creator9/41
  Init2/42(vc1ss) -> Bus Creator9/42
  Init2/43(vc2ss) -> Bus Creator9/43
  Init2/44(vc3ss) -> Bus Creator9/44
  Init2/45(vc4ss) -> Bus Creator9/45
  Init2/46(ilt0ss) -> Bus Creator9/46
  Init2/47(ilt1ss) -> Bus Creator9/47
  Init2/48(ilt2ss) -> Bus Creator9/48
  Init2/49(ilt3ss) -> Bus Creator9/49
  Init2/50(ilt4ss) -> Bus Creator9/50
  Init/1(E0) -> Bus Creator2/1
  Init/2(E1) -> Bus Creator2/2
  Init/3(E2) -> Bus Creator2/3
  Init/4(E3) -> Bus Creator2/4
  Init/5(E4) -> Bus Creator2/5
  Init/6(U0) -> Bus Creator2/6
  Init/7(U1) -> Bus Creator2/7
  Init/8(U2) -> Bus Creator2/8
  Init/9(U3) -> Bus Creator2/9
  Init/10(U4) -> Bus Creator2/10
  Init/11(R1t0) -> Bus Creator2/11
  Init/12(R1t1) -> Bus Creator2/12
  Init/13(R1t2) -> Bus Creator2/13
  Init/14(R1t3) -> Bus Creator2/14
  Init/15(R1t4) -> Bus Creator2/15
  Init/16(R2t0) -> Bus Creator2/16
  Init/17(R2t1) -> Bus Creator2/17
  Init/18(R2t2) -> Bus Creator2/18
  Init/19(R2t3) -> Bus Creator2/19
  Init/20(R2t4) -> Bus Creator2/20
  Init/21(C0) -> Bus Creator2/21
  Init/22(C1) -> Bus Creator2/22
  Init/23(C2) -> Bus Creator2/23
  Init/24(C3) -> Bus Creator2/24
  Init/25(C4) -> Bus Creator2/25
  Init/26(L0) -> Bus Creator2/26
  Init/27(L1) -> Bus Creator2/27
  Init/28(L2) -> Bus Creator2/28
  Init/29(L3) -> Bus Creator2/29
  Init/30(L4) -> Bus Creator2/30
  Init/31(Lt0) -> Bus Creator2/31
  Init/32(Lt1) -> Bus Creator2/32
  Init/33(Lt2) -> Bus Creator2/33
  Init/34(Lt3) -> Bus Creator2/34
  Init/35(Lt4) -> Bus Creator2/35
  Init/36(Rab) -> Bus Creator2/36
  Init/37(Lab) -> Bus Creator2/37
  Init/38(Rac) -> Bus Creator2/38
  Init/39(Lac) -> Bus Creator2/39
  Init/40(il0d) -> Bus Creator2/40
  Init/41(il1d) -> Bus Creator2/41
  Init/42(il2d) -> Bus Creator2/42
  Init/43(il3d) -> Bus Creator2/43
  Init/44(il4d) -> Bus Creator2/44
  Init/45(vc0ss) -> Bus Creator2/45
  Init/46(vc1ss) -> Bus Creator2/46
  Init/47(vc2ss) -> Bus Creator2/47
  Init/48(vc3ss) -> Bus Creator2/48
  Init/49(vc4ss) -> Bus Creator2/49
  Init/50(ilt0ss) -> Bus Creator2/50
  Init/51(ilt1ss) -> Bus Creator2/51
  Init/52(ilt2ss) -> Bus Creator2/52
  Init/53(ilt3ss) -> Bus Creator2/53
  Init/54(ilt4ss) -> Bus Creator2/54
  Init/55(iabss) -> whole_sys/74(iabd), Bus Creator2/55
  Init/56(iacss) -> whole_sys/75(iacd), Bus Creator2/56
  whole_sys/17(iacdot) -> ilt6/1
  whole_sys/16(iabdot) -> ilt8/1
  whole_sys/15(ilt4dot) -> ilt4/1
  whole_sys/14(ilt3dot) -> ilt3/1
  whole_sys/13(ilt2dot) -> ilt2/1
  whole_sys/12(ilt1dot) -> ilt1/1
  whole_sys/11(ilt0dot) -> ilt0/1
  whole_sys/10(vc4dot) -> vc4/1
  whole_sys/9(vc3dot) -> vc3/1
  whole_sys/8(vc2dot) -> vc2/1
  whole_sys/7(vc1dot) -> vc1/1
  whole_sys/6(vc0dot) -> vc0/1
  whole_sys/5(il4dot) -> il4/1
  whole_sys/4(il3dot) -> il3/1
  whole_sys/3(il2dot) -> il2/1
  whole_sys/2(il1dot) -> il1/1
  whole_sys/1(il0dot) -> il0/1
  Bus Selector21/1 -> utt/1(E0)  "<E0>"
  Bus Selector21/2 -> utt/2(E1)  "<E1>"
  Bus Selector21/3 -> utt/3(E2)  "<E2>"
  Bus Selector21/4 -> utt/4(E3)  "<E3>"
  Bus Selector21/5 -> utt/5(E4)  "<E4>"
  Bus Selector21/6 -> utt/6(il0d)  "<il0d>"
  Bus Selector21/7 -> utt/7(il1d)  "<il1d>"
  Bus Selector21/8 -> utt/8(il2d)  "<il2d>"
  Bus Selector21/9 -> utt/9(il3d)  "<il3d>"
  Bus Selector21/10 -> utt/10(il4d)  "<il4d>"
  il0/1 -> Bus Creator1/1
  il1/1 -> Bus Creator1/2
  il2/1 -> Bus Creator1/3
  il3/1 -> Bus Creator1/4
  il4/1 -> Bus Creator1/5
  vc0/1 -> Bus Creator1/6
  vc2/1 -> Bus Creator1/8
  vc3/1 -> Bus Creator1/9
  vc4/1 -> Bus Creator1/10
  ilt0/1 -> Bus Creator1/11
  ilt1/1 -> Bus Creator1/12
  ilt2/1 -> Bus Creator1/13
  ilt3/1 -> Bus Creator1/14
  ilt4/1 -> Bus Creator1/15
  ilt8/1 -> Bus Creator1/16, whole_sys1/56(iab)
  ilt6/1 -> whole_sys2/56(iac), Bus Creator1/17
  Bus Selector22/1 -> utt/11(il0)  "<signal1>"
  Bus Selector22/2 -> utt/12(il1)  "<signal2>"
  Bus Selector22/3 -> utt/13(il2)  "<signal3>"
  Bus Selector22/4 -> utt/14(il3)  "<signal4>"
  Bus Selector22/5 -> utt/15(il4)  "<signal5>"
  Bus Selector23/1 -> utt/16(vc0d)  "<signal1>"
  Bus Selector23/2 -> utt/17(vc1d)  "<signal2>"
  Bus Selector23/3 -> utt/18(vc2d)  "<signal3>"
  Bus Selector23/4 -> utt/19(vc3d)  "<signal4>"
  Bus Selector23/5 -> utt/20(vc4d)  "<signal5>"
  cont/1(vc0d-) -> Bus Creator10/1
  cont/2(vc1d-) -> Bus Creator10/2
  cont/3(vc2d-) -> Bus Creator10/3
  cont/4(vc3d-) -> Bus Creator10/4
  cont/5(vc4d-) -> Bus Creator10/5
  cont/11(iabd-) -> cont1/41(iabd), Bus Creator10/6
  Bus Creator10/1 -> Bus Selector23/1
  Bus Selector24/1 -> cont/6(R1t0)  "<R1t0>"
  Bus Selector24/2 -> cont/7(R1t1)  "<R1t1>"
  Bus Selector24/3 -> cont/8(R1t2)  "<R1t2>"
  Bus Selector24/4 -> cont/9(R1t3)  "<R1t3>"
  Bus Selector24/5 -> cont/10(R1t4)  "<R1t4>"
  Bus Selector24/6 -> cont/11(R2t0)  "<R2t0>"
  Bus Selector24/7 -> cont/12(R2t1)  "<R2t1>"
  Bus Selector24/8 -> cont/13(R2t2)  "<R2t2>"
  Bus Selector24/9 -> cont/14(R2t3)  "<R2t3>"
  Bus Selector24/10 -> cont/15(R2t4)  "<R2t4>"
  Bus Selector24/11 -> cont/16(il0d)  "<il0d>"
  Bus Selector24/12 -> cont/17(il1d)  "<il1d>"
  Bus Selector24/13 -> cont/18(il2d)  "<il2d>"
  Bus Selector24/14 -> cont/19(il3d)  "<il3d>"
  Bus Selector24/15 -> cont/20(il4d)  "<il4d>"
  Bus Selector24/16 -> cont/21(C0)  "<C0>"
  Bus Selector24/17 -> cont/22(C1)  "<C1>"
  Bus Selector24/18 -> cont/23(C2)  "<C2>"
  Bus Selector24/19 -> cont/24(C3)  "<C3>"
  Bus Selector24/20 -> cont/25(C4)  "<C4>"
  Bus Selector24/21 -> cont/26(Lt0)  "<Lt0>"
  Bus Selector24/22 -> cont/27(Lt1)  "<Lt1>"
  Bus Selector24/23 -> cont/28(Lt2)  "<Lt2>"
  Bus Selector24/24 -> cont/29(Lt3)  "<Lt3>"
  Bus Selector24/25 -> cont/30(Lt4)  "<Lt4>"
  Bus Selector24/26 -> cont/31(vc0ss)  "<vc0ss>"
  Bus Selector24/27 -> cont/32(vc1ss)  "<vc1ss>"
  Bus Selector24/28 -> cont/33(vc2ss)  "<vc2ss>"
  Bus Selector24/29 -> cont/34(vc3ss)  "<vc3ss>"
  Bus Selector24/30 -> cont/35(vc4ss)  "<vc4ss>"
  Bus Selector24/31 -> cont/36(ilt0ss)  "<ilt0ss>"
  Bus Selector24/32 -> cont/37(ilt1ss)  "<ilt1ss>"
  Bus Selector24/33 -> cont/38(ilt2ss)  "<ilt2ss>"
  Bus Selector24/34 -> cont/39(ilt3ss)  "<ilt3ss>"
  Bus Selector24/35 -> cont/40(ilt4ss)  "<ilt4ss>"
  Bus Selector24/36 -> cont/41(Lab)  "<Lab>"
  Bus Selector24/37 -> cont/42(Lac)  "<Lac>"
  Bus Selector24/38 -> cont/43(Rab)  "<Rab>"
  Bus Selector24/39 -> cont/44(Rac)  "<Rac>"
  Bus Selector24/40 -> cont/45(iabss)  "<iabss>"
  Bus Selector24/41 -> cont/46(iacss)  "<iacss>"
  utt/1(ut0-) -> Switch6/1, cont/1(ut0)
  utt/2(ut1) -> Switch5/1, cont/2(ut1)
  utt/3(ut2) -> cont/3(ut2), Switch7/1
  utt/4(ut3) -> cont/4(ut3), Switch8/1
  utt/5(ut4) -> Switch9/1, cont/5(ut4)
  Ralpha/1 -> utt/21(Ralp)
  Rbeta/1 -> utt/22(Rbeta)
  Rgamma/1 -> utt/23(Rgamma)
  Rdelta/1 -> utt/24(Rdelta)
  Reta/1 -> utt/25(Reta)
  Rgamma1/1 -> utt1/23(Rgamma)
  Rbeta1/1 -> utt1/22(Rbeta)
  Rdelta1/1 -> utt1/24(Rdelta)
  Reta1/1 -> utt1/25(Reta)
  Ralpha1/1 -> utt1/21(Ralp)
  Ralpha2/1 -> utt2/21(Ralp)
  Rbeta2/1 -> utt2/22(Rbeta)
  Rgamma2/1 -> utt2/23(Rgamma)
  Rdelta2/1 -> utt2/24(Rdelta)
  Reta2/1 -> utt2/25(Reta)
  utt2/1(ut0-) -> Switch11/1, cont2/1(ut0)
  utt2/2(ut1) -> Switch10/1, cont2/2(ut1)
  utt2/3(ut2) -> cont2/3(ut2), Switch12/1
  utt2/4(ut3) -> Switch13/1, cont2/4(ut3)
  utt2/5(ut4) -> Switch14/1, cont2/5(ut4)
  Bus Selector25/1 -> utt1/1(E0)  "<E0>"
  Bus Selector25/2 -> utt1/2(E1)  "<E1>"
  Bus Selector25/3 -> utt1/3(E2)  "<E2>"
  Bus Selector25/4 -> utt1/4(E3)  "<E3>"
  Bus Selector25/5 -> utt1/5(E4)  "<E4>"
  Bus Selector25/6 -> utt1/6(il0d)  "<il0d>"
  Bus Selector25/7 -> utt1/7(il1d)  "<il1d>"
  Bus Selector25/8 -> utt1/8(il2d)  "<il2d>"
  Bus Selector25/9 -> utt1/9(il3d)  "<il3d>"
  Bus Selector25/10 -> utt1/10(il4d)  "<il4d>"
  Bus Selector26/1 -> utt1/11(il0)  "<signal1>"
  Bus Selector26/2 -> utt1/12(il1)  "<signal2>"
  Bus Selector26/3 -> utt1/13(il2)  "<signal3>"
  Bus Selector26/4 -> utt1/14(il3)  "<signal4>"
  Bus Selector26/5 -> utt1/15(il4)  "<signal5>"
  cont1/2(vc1d-) -> utt1/17(vc1d)
  cont1/3(vc2d-) -> utt1/18(vc2d)
  cont1/4(vc3d-) -> utt1/19(vc3d)
  cont1/5(vc4d-) -> utt1/20(vc4d)
  cont1/6(ilt0d-) -> ?
  cont1/7(ilt1d-) -> ?
  utt1/1(ut0-) -> Switch1/1, cont1/1(ut0)
  utt1/2(ut1) -> Switch/1, cont1/2(ut1)
  utt1/3(ut2) -> Switch2/1, cont1/3(ut2)
  utt1/4(ut3) -> Switch3/1, cont1/4(ut3)
  utt1/5(ut4) -> Switch4/1, cont1/5(ut4)
  Bus Selector28/1 -> cont1/6(R1t0)  "<R1t0>"
  Bus Selector28/2 -> cont1/7(R1t1)  "<R1t1>"
  Bus Selector28/3 -> cont1/8(R1t2)  "<R1t2>"
  Bus Selector28/4 -> cont1/9(R1t3)  "<R1t3>"
  Bus Selector28/5 -> cont1/10(R1t4)  "<R1t4>"
  Bus Selector28/6 -> cont1/11(R2t0)  "<R2t0>"
  Bus Selector28/7 -> cont1/12(R2t1)  "<R2t1>"
  Bus Selector28/8 -> cont1/13(R2t2)  "<R2t2>"
  Bus Selector28/9 -> cont1/14(R2t3)  "<R2t3>"
  Bus Selector28/10 -> cont1/15(R2t4)  "<R2t4>"
  Bus Selector28/11 -> cont1/16(il0d)  "<il0d>"
  Bus Selector28/12 -> cont1/17(il1d)  "<il1d>"
  Bus Selector28/13 -> cont1/18(il2d)  "<il2d>"
  Bus Selector28/14 -> cont1/19(il3d)  "<il3d>"
  Bus Selector28/15 -> cont1/20(il4d)  "<il4d>"
  Bus Selector28/16 -> cont1/21(C0)  "<C0>"
  Bus Selector28/17 -> cont1/22(C1)  "<C1>"
  Bus Selector28/18 -> cont1/23(C2)  "<C2>"
  Bus Selector28/19 -> cont1/24(C3)  "<C3>"
  Bus Selector28/20 -> cont1/25(C4)  "<C4>"
  Bus Selector28/21 -> cont1/26(Lt0)  "<Lt0>"
  Bus Selector28/22 -> cont1/27(Lt1)  "<Lt1>"
  Bus Selector28/23 -> cont1/28(Lt2)  "<Lt2>"
  Bus Selector28/24 -> cont1/29(Lt3)  "<Lt3>"
  Bus Selector28/25 -> cont1/30(Lt4)  "<Lt4>"
  Bus Selector28/26 -> cont1/31(vc0ss)  "<vc0ss>"
  Bus Selector28/27 -> cont1/32(vc1ss)  "<vc1ss>"
  Bus Selector28/28 -> cont1/33(vc2ss)  "<vc2ss>"
  Bus Selector28/29 -> cont1/34(vc3ss)  "<vc3ss>"
  Bus Selector28/30 -> cont1/35(vc4ss)  "<vc4ss>"
  Bus Selector28/31 -> cont1/36(ilt0ss)  "<ilt0ss>"
  Bus Selector28/32 -> cont1/37(ilt1ss)  "<ilt1ss>"
  Bus Selector28/33 -> cont1/38(ilt2ss)  "<ilt2ss>"
  Bus Selector28/34 -> cont1/39(ilt3ss)  "<ilt3ss>"
  Bus Selector28/35 -> cont1/40(ilt4ss)  "<ilt4ss>"
  Bus Selector29/1 -> cont2/6(R1t0)  "<R1t0>"
  Bus Selector29/2 -> cont2/7(R1t1)  "<R1t1>"
  Bus Selector29/3 -> cont2/8(R1t2)  "<R1t2>"
  Bus Selector29/4 -> cont2/9(R1t3)  "<R1t3>"
  Bus Selector29/5 -> cont2/10(R1t4)  "<R1t4>"
  Bus Selector29/6 -> cont2/11(R2t0)  "<R2t0>"
  Bus Selector29/7 -> cont2/12(R2t1)  "<R2t1>"
  Bus Selector29/8 -> cont2/13(R2t2)  "<R2t2>"
  Bus Selector29/9 -> cont2/14(R2t3)  "<R2t3>"
  Bus Selector29/10 -> cont2/15(R2t4)  "<R2t4>"
  Bus Selector29/11 -> cont2/16(il0d)  "<il0d>"
  Bus Selector29/12 -> cont2/17(il1d)  "<il1d>"
  Bus Selector29/13 -> cont2/18(il2d)  "<il2d>"
  Bus Selector29/14 -> cont2/19(il3d)  "<il3d>"
  Bus Selector29/15 -> cont2/20(il4d)  "<il4d>"
  Bus Selector29/16 -> cont2/21(C0)  "<C0>"
  Bus Selector29/17 -> cont2/22(C1)  "<C1>"
  Bus Selector29/18 -> cont2/23(C2)  "<C2>"
  Bus Selector29/19 -> cont2/24(C3)  "<C3>"
  Bus Selector29/20 -> cont2/25(C4)  "<C4>"
  Bus Selector29/21 -> cont2/26(Lt0)  "<Lt0>"
  Bus Selector29/22 -> cont2/27(Lt1)  "<Lt1>"
  Bus Selector29/23 -> cont2/28(Lt2)  "<Lt2>"
  Bus Selector29/24 -> cont2/29(Lt3)  "<Lt3>"
  Bus Selector29/25 -> cont2/30(Lt4)  "<Lt4>"
  Bus Selector29/26 -> cont2/31(vc0ss)  "<vc0ss>"
  Bus Selector29/27 -> cont2/32(vc1ss)  "<vc1ss>"
  Bus Selector29/28 -> cont2/33(vc2ss)  "<vc2ss>"
  Bus Selector29/29 -> cont2/34(vc3ss)  "<vc3ss>"
  Bus Selector29/30 -> cont2/35(vc4ss)  "<vc4ss>"
  Bus Selector29/31 -> cont2/36(ilt0ss)  "<ilt0ss>"
  Bus Selector29/32 -> cont2/37(ilt1ss)  "<ilt1ss>"
  Bus Selector29/33 -> cont2/38(ilt2ss)  "<ilt2ss>"
  Bus Selector29/34 -> cont2/39(ilt3ss)  "<ilt3ss>"
  Bus Selector29/35 -> cont2/40(ilt4ss)  "<ilt4ss>"
  cont/12(iacd-) -> cont2/41(iacd), Bus Creator10/7
  Bus Selector1/1 -> whole_sys1/6(E0)  "<E0>"
  Bus Selector1/2 -> whole_sys1/7(E1)  "<E1>"
  Bus Selector1/3 -> whole_sys1/8(E2)  "<E2>"
  Bus Selector1/4 -> whole_sys1/9(E3)  "<E3>"
  Bus Selector1/5 -> whole_sys1/10(E4)  "<E4>"
  Bus Selector1/6 -> whole_sys1/11(R1t0)  "<R1t0>"
  Bus Selector1/7 -> whole_sys1/12(R1t1)  "<R1t1>"
  Bus Selector1/8 -> whole_sys1/13(R1t2)  "<R1t2>"
  Bus Selector1/9 -> whole_sys1/14(R1t3)  "<R1t3>"
  Bus Selector1/10 -> whole_sys1/15(R1t4)  "<R1t4>"
  Bus Selector1/11 -> whole_sys1/16(R2t0)  "<R2t0>"
  Bus Selector1/12 -> whole_sys1/17(R2t1)  "<R2t1>"
  Bus Selector1/13 -> whole_sys1/18(R2t2)  "<R2t2>"
  Bus Selector1/14 -> whole_sys1/19(R2t3)  "<R2t3>"
  Bus Selector1/15 -> whole_sys1/20(R2t4)  "<R2t4>"
  Bus Selector1/16 -> whole_sys1/21(C0)  "<C0>"
  Bus Selector1/17 -> whole_sys1/22(C1)  "<C1>"
  Bus Selector1/18 -> whole_sys1/23(C2)  "<C2>"
  Bus Selector1/19 -> whole_sys1/24(C3)  "<C3>"
  Bus Selector1/20 -> whole_sys1/25(C4)  "<C4>"
  Bus Selector1/21 -> whole_sys1/26(L0)  "<L0>"
  Bus Selector1/22 -> whole_sys1/27(L1)  "<L1>"
  Bus Selector1/23 -> whole_sys1/28(L2)  "<L2>"
  Bus Selector1/24 -> whole_sys1/29(L3)  "<L3>"
  Bus Selector1/25 -> whole_sys1/30(L4)  "<L4>"
  Bus Selector1/26 -> whole_sys1/31(Lt0)  "<Lt0>"
  Bus Selector1/27 -> whole_sys1/32(Lt1)  "<Lt1>"
  Bus Selector1/28 -> whole_sys1/33(Lt2)  "<Lt2>"
  Bus Selector1/29 -> whole_sys1/34(Lt3)  "<Lt3>"
  Bus Selector1/30 -> whole_sys1/35(Lt4)  "<Lt4>"
  Bus Selector1/31 -> whole_sys1/36(il0d)  "<il0d>"
  Bus Selector1/32 -> whole_sys1/37(il1d)  "<il1d>"
  Bus Selector1/33 -> whole_sys1/38(il2d)  "<il2d>"
  Bus Selector1/34 -> whole_sys1/39(il3d)  "<il3d>"
  Bus Selector1/35 -> whole_sys1/40(il4d)  "<il4d>"
  Bus Selector6/1 -> whole_sys1/41(il0)  "<signal1>"
  Bus Selector6/2 -> whole_sys1/42(il1)  "<signal2>"
  Bus Selector6/3 -> whole_sys1/43(il2)  "<signal3>"
  Bus Selector6/4 -> whole_sys1/44(il3)  "<signal4>"
  Bus Selector6/5 -> whole_sys1/45(il4)  "<signal5>"
  Bus Selector6/6 -> whole_sys1/46(vc0)  "<signal6>"
  Bus Selector6/7 -> whole_sys1/47(vc1)  "<signal7>"
  Bus Selector6/8 -> whole_sys1/48(vc2)  "<signal8>"
  Bus Selector6/9 -> whole_sys1/49(vc3)  "<signal9>"
  Bus Selector6/10 -> whole_sys1/50(vc4)  "<signal10>"
  Bus Selector6/11 -> whole_sys1/51(ilt0)  "<signal11>"
  Bus Selector6/12 -> whole_sys1/52(ilt1)  "<signal12>"
  Bus Selector6/13 -> whole_sys1/53(ilt2)  "<signal13>"
  Bus Selector6/14 -> whole_sys1/54(ilt3)  "<signal14>"
  Bus Selector6/15 -> whole_sys1/55(ilt4)  "<signal15>"
  Bus Selector8/1 -> whole_sys1/57(vc0d)  "<vc0ss>"
  Bus Selector8/2 -> whole_sys1/58(vc1d)  "<vc1ss>"
  Bus Selector8/3 -> whole_sys1/59(vc2d)  "<vc2ss>"
  Bus Selector8/4 -> whole_sys1/60(vc3d)  "<vc3ss>"
  Bus Selector8/5 -> whole_sys1/61(vc4d)  "<vc4ss>"
  Bus Selector8/6 -> whole_sys1/62(ilt0d)  "<ilt0ss>"
  Bus Selector8/7 -> whole_sys1/63(ilt1d)  "<ilt1ss>"
  Bus Selector8/8 -> whole_sys1/64(ilt2d)  "<ilt2ss>"
  Bus Selector8/9 -> whole_sys1/65(ilt3d)  "<ilt3ss>"
  Bus Selector8/10 -> whole_sys1/66(ilt4d)  "<ilt4ss>"
  Bus Selector30/1 -> utt2/1(E0)  "<E0>"
  Bus Selector30/2 -> utt2/2(E1)  "<E1>"
  Bus Selector30/3 -> utt2/3(E2)  "<E2>"
  Bus Selector30/4 -> utt2/4(E3)  "<E3>"
  Bus Selector30/5 -> utt2/5(E4)  "<E4>"
  Bus Selector30/6 -> utt2/6(il0d)  "<il0d>"
  Bus Selector30/7 -> utt2/7(il1d)  "<il1d>"
  Bus Selector30/8 -> utt2/8(il2d)  "<il2d>"
  Bus Selector30/9 -> utt2/9(il3d)  "<il3d>"
  Bus Selector30/10 -> utt2/10(il4d)  "<il4d>"
  Bus Selector31/1 -> utt2/11(il0)  "<signal1>"
  Bus Selector31/2 -> utt2/12(il1)  "<signal2>"
  Bus Selector31/3 -> utt2/13(il2)  "<signal3>"
  Bus Selector31/4 -> utt2/14(il3)  "<signal4>"
  Bus Selector31/5 -> utt2/15(il4)  "<signal5>"
  cont2/1(vc0d-) -> utt2/16(vc0d)
  cont2/2(vc1d-) -> utt2/17(vc1d)
  cont2/3(vc2d-) -> utt2/18(vc2d)
  cont2/4(vc3d-) -> utt2/19(vc3d)
  cont2/5(vc4d-) -> utt2/20(vc4d)
  Switch1/1 -> Bus Creator13/1, PWM5/1(D)
  Switch/1 -> Bus Creator13/2, PWM6/1(D)
  Switch2/1 -> Bus Creator13/3, PWM7/1(D)
  Switch3/1 -> Bus Creator13/4, PWM8/1(D)
  Switch4/1 -> Bus Creator13/5, PWM9/1(D)
  Switch5/1 -> Bus Creator12/2, PWM1/1(D)
  Switch6/1 -> Bus Creator12/1, PWM0/1(D)
  Switch7/1 -> Bus Creator12/3, PWM2/1(D)
  Switch8/1 -> Bus Creator12/4, PWM3/1(D)
  Switch9/1 -> Bus Creator12/5, PWM4/1(D)
  Switch11/1 -> Bus Creator14/1, PWM10/1(D)
  Switch10/1 -> Bus Creator14/2, PWM11/1(D)
  Switch12/1 -> Bus Creator14/3, PWM12/1(D)
  Switch13/1 -> Bus Creator14/4, PWM13/1(D)
  Switch14/1 -> Bus Creator14/5, PWM14/1(D)
  Bus Selector36/1 -> Saturation5/1  "<U0>"
  Bus Selector36/2 -> Saturation6/1  "<U1>"
  Bus Selector36/3 -> Saturation7/1  "<U2>"
  Bus Selector36/4 -> Saturation8/1  "<U3>"
  Bus Selector36/5 -> Saturation9/1  "<U4>"
  Bus Selector37/1 -> Saturation10/1  "<U0>"
  Bus Selector37/2 -> Saturation11/1  "<U1>"
  Bus Selector37/3 -> Saturation12/1  "<U2>"
  Bus Selector37/4 -> Saturation13/1  "<U3>"
  Bus Selector37/5 -> Saturation14/1  "<U4>"
  Saturation/1 -> Switch6/3
  Saturation1/1 -> Switch5/3
  Saturation2/1 -> Switch7/3
  Saturation3/1 -> Switch8/3
  Saturation4/1 -> Switch9/3
  Saturation14/1 -> Switch14/3
  Saturation10/1 -> Switch11/3
  Saturation11/1 -> Switch10/3
  Saturation12/1 -> Switch12/3
  Saturation13/1 -> Switch13/3
  Saturation5/1 -> Switch1/3
  Saturation6/1 -> Switch/3
  Saturation7/1 -> Switch2/3
  Saturation8/1 -> Switch3/3
  Saturation9/1 -> Switch4/3
  "nocontrol "/1 -> " Switch"/2
  Init1/41(vc0ss) -> Bus Creator8/41
  cont1/1(vc0d-) -> utt1/16(vc0d)
  vc1/1 -> Bus Creator1/7
  vc5/1 -> whole_sys/62(vc0b), Bus Creator3/6
  PWM9/1(P) -> whole_sys1/5(u4)
  Bus Selector27/1 -> il15/1  "<signal1>"
  Bus Selector27/3 -> il15/3  "<signal3>"
  Bus Selector27/4 -> il15/4  "<signal4>"
  Bus Selector27/5 -> il15/5  "<signal5>"
  Bus Selector27/6 -> vc6/1  "<signal6>"
  Bus Selector27/8 -> vc6/3  "<signal8>"
  Bus Selector27/9 -> vc6/4  "<signal9>"
  Bus Selector27/10 -> vc6/5  "<signal10>"
  Bus Selector27/12 -> ilt7/2  "<signal12>"
  Bus Selector27/11 -> ilt7/1  "<signal11>"
  Bus Selector27/13 -> ilt7/3  "<signal13>"
  Bus Selector27/14 -> ilt7/4  "<signal14>"
  Bus Selector27/15 -> ilt7/5  "<signal15>"
  Bus Selector27/2 -> il15/2  "<signal2>"
  Bus Selector27/7 -> vc6/2  "<signal7>"
  Bus Selector32/1 -> il16/1  "<signal1>"
  Bus Selector32/3 -> il16/3  "<signal3>"
  Bus Selector32/4 -> il16/4  "<signal4>"
  Bus Selector32/5 -> il16/5  "<signal5>"
  Bus Selector32/6 -> vc10/1  "<signal6>"
  Bus Selector32/8 -> vc10/3  "<signal8>"
  Bus Selector32/9 -> vc10/4  "<signal9>"
  Bus Selector32/10 -> vc10/5  "<signal10>"
  Bus Selector32/12 -> ilt21/2  "<signal12>"
  Bus Selector32/11 -> ilt21/1  "<signal11>"
  Bus Selector32/13 -> ilt21/3  "<signal13>"
  Bus Selector32/14 -> ilt21/4  "<signal14>"
  Bus Selector32/15 -> ilt21/5  "<signal15>"
  Bus Selector32/2 -> il16/2  "<signal2>"
  Bus Selector32/7 -> vc10/2  "<signal7>"
  Bus Selector39/1 -> he3/1  "<signal16>"
  Bus Selector39/2 -> he3/2  "<signal17>"
  MATLAB Function/1(Ea0) -> Bus Creator11/1
  MATLAB Function/2(Ea1) -> Bus Creator11/2
  MATLAB Function/3(Eb0) -> Bus Creator11/3
  MATLAB Function/4(Ec0) -> Bus Creator11/4
  MATLAB Function/5(Rab) -> Bus Creator11/5
  MATLAB Function/6(Rac) -> Bus Creator11/6
  Bus Creator11/1 -> Bus Selector33/1, Bus Selector34/1, Bus Selector35/1
  Bus Selector35/1 -> Init/1("Rab ")  "<Rab>"
  Bus Selector35/2 -> Init/2("Rac ")  "<Rac>"
  Bus Selector35/3 -> Init/3("E0 ")  "<Ea0>"
  Bus Selector35/4 -> Init/4("E1 ")  "<Ea1>"
  Bus Selector35/5 -> Init/5(Eb)  "<Eb0>"
  Bus Selector35/6 -> Init/6(Ec)  "<Ec0>"
  Bus Selector33/1 -> Init1/1("E0 ")  "<Eb0>"
  Bus Selector33/2 -> Init1/2(Rab)  "<Rab>"
  Bus Selector33/3 -> Init1/3(Ea0)  "<Ea0>"
  Bus Selector34/1 -> Init2/1("E0 ")  "<Ec0>"
  Bus Selector34/2 -> Init2/3(Rac)  "<Rac>"
  Bus Selector34/3 -> Init2/2(Ea1)  "<Ea1>"
  " Switch"/1 -> Scope4/1, Switch4/2, Switch3/2, Switch2/2, Switch/2, Switch1/2, Switch14/2, Switch13/2, Switch12/2, Switch10/2, Switch11/2, Switch9/2, Switch8/2, Switch7/2, Switch5/2, Switch6/2
  Bus Creator7/1 -> Bus Selector40/1, Bus Selector17/1, Bus Selector19/1
  Bus Selector38/1 -> il0_file5/1  "<signal1>"
  Bus Selector38/2 -> il1_file2/1  "<signal2>"
  Bus Selector38/3 -> il2_file6/1  "<signal3>"
  Bus Selector40/1 -> he0_file3/1  "<He0>"
  Bus Selector40/2 -> he1_file3/1  "<He1>"
  Bus Selector40/3 -> he2_file1/1  "<He2>"
  Bus Creator5/1 -> Bus Selector32/1, Bus Selector38/1, Bus Selector7/1, Bus Selector31/1
  Bus Selector38/4 -> il2_file7/1  "<signal4>"
  Bus Selector38/5 -> il2_file8/1  "<signal5>"
  Bus Selector38/6 -> il0_file6/1  "<signal6>"
  Bus Selector38/7 -> vc1_file1/1  "<signal7>"
  Bus Selector38/8 -> vc2_file1/1  "<signal8>"
  Bus Selector38/9 -> il0_file7/1  "<signal9>"
  Bus Selector38/10 -> il0_file8/1  "<signal10>"
  Bus Selector38/11 -> ilt0_file3/1  "<signal11>"
  Bus Selector38/12 -> ilt1_file1/1  "<signal12>"
  Bus Selector38/13 -> ilt2_file1/1  "<signal13>"
  Bus Selector38/14 -> ilt0_file5/1  "<signal14>"
  Bus Selector38/15 -> ilt0_file4/1  "<signal15>"
  Bus Selector40/4 -> he_file7/1  "<He3>"
  Bus Selector40/5 -> he_file8/1  "<He4>"
  Bus Selector40/6 -> he_file4/1  "<He>"
  Bus Selector40/7 -> he_file6/1  "<H>"
  Bus Selector40/8 -> he0_file5/1  "<H0>"
  Bus Selector40/9 -> he1_file4/1  "<H1>"
  Bus Selector40/10 -> he1_file5/1  "<H2>"
  Bus Selector40/11 -> he0_file4/1  "<H3>"
  Bus Selector40/12 -> he0_file6/1  "<H4>"
  Bus Selector15/1 -> ilt5/1  "<signal1>"
  Bus Selector15/2 -> ilt5/2  "<signal2>"
  Bus Selector15/3 -> ilt5/3  "<signal3>"
  Bus Selector15/4 -> ilt5/4  "<signal4>"
  Bus Selector15/5 -> ilt5/5  "<signal5>"
  Bus Selector16/1 -> il0_file4/1  "<signal1>"
  Bus Selector16/2 -> il1_file1/1  "<signal2>"
  Bus Selector16/3 -> il2_file3/1  "<signal3>"
  Bus Selector16/4 -> il2_file5/1  "<signal4>"
  Bus Selector16/5 -> il2_file4/1  "<signal5>"
  Bus Creator12/1 -> Bus Selector15/1, Bus Selector46/1
  Bus Selector18/1 -> il0_file1/1  "<signal1>"
  Bus Selector18/2 -> il1_file3/1  "<signal2>"
  Bus Selector18/3 -> il2_file1/1  "<signal3>"
  Bus Selector18/4 -> il2_file9/1  "<signal4>"
  Bus Selector18/5 -> il2_file2/1  "<signal5>"
  Bus Selector41/2 -> he1_file9/1  "<E1>"
  Bus Selector41/1 -> he0_file1/1  "<E0>"
  Bus Selector41/3 -> he1_file10/1  "<E2>"
  Bus Selector41/4 -> he1_file11/1  "<E3>"
  Bus Selector41/5 -> he1_file12/1  "<E4>"
  Bus Selector41/6 -> he0_file2/1  "<R2t0>"
  Bus Selector41/7 -> he1_file16/1  "<R2t1>"
  Bus Selector41/8 -> he1_file13/1  "<R2t2>"
  Bus Selector41/9 -> he1_file14/1  "<R2t3>"
  Bus Selector41/10 -> he1_file15/1  "<R2t4>"
  Band-Limited White Noise/1 -> MATLAB Function/1(m0), Init/7(m0), Scope1/2
  Band-Limited White Noise1/1 -> MATLAB Function/2(m1), Init1/4(m1)
  Band-Limited White Noise2/1 -> MATLAB Function/3(m2), Init2/4(m2)
  Bus Selector42/2 -> ilt22/2  "<E1>"
  Bus Selector42/3 -> ilt22/3  "<E2>"
  Bus Selector42/4 -> ilt22/4  "<E3>"
  Bus Selector42/5 -> ilt22/5  "<E4>"
  Bus Creator2/1 -> Bus Selector2/1, Bus Selector4/1, Bus Selector45/1, Bus Selector42/1, Bus Selector10/1, Bus Selector21/1, Bus Selector24/1
  Bus Selector43/1 -> ilt23/1  "<signal1>"
  Bus Selector43/2 -> ilt23/2  "<signal2>"
  Bus Selector43/3 -> ilt23/3  "<signal3>"
  Bus Selector43/4 -> ilt23/4  "<signal4>"
  Bus Selector43/5 -> ilt23/5  "<signal5>"
  Bus Selector44/1 -> ilt24/1  "<signal1>"
  Bus Selector44/2 -> ilt24/2  "<signal2>"
  Bus Selector44/3 -> ilt24/3  "<signal3>"
  Bus Selector44/4 -> ilt24/4  "<signal4>"
  Bus Selector44/5 -> ilt24/5  "<signal5>"
  Bus Creator8/1 -> Bus Selector36/1, Bus Selector1/1, Bus Selector28/1, Bus Selector25/1, Bus Selector8/1
  Bus Creator9/1 -> Bus Selector29/1, Bus Selector37/1, Bus Selector5/1, Bus Selector20/1, Bus Selector30/1
  Bus Selector42/1 -> ilt22/1  "<E0>"
  Bus Creator13/1 -> Bus Selector43/1, Bus Selector16/1
  Bus Creator14/1 -> Bus Selector44/1, Bus Selector18/1
  Bus Selector45/1 -> he0_file10/1  "<E0>"
  Bus Selector45/2 -> he1_file27/1  "<E1>"
  Bus Selector45/3 -> he1_file24/1  "<E2>"
  Bus Selector45/4 -> he1_file25/1  "<E3>"
  Bus Selector45/5 -> he1_file26/1  "<E4>"
  Bus Selector46/1 -> il0_file2/1  "<signal1>"
  Bus Selector46/2 -> il1_file4/1  "<signal2>"
  Bus Selector46/3 -> il2_file10/1  "<signal3>"
  Bus Selector46/4 -> il2_file12/1  "<signal4>"
  Bus Selector46/5 -> il2_file11/1  "<signal5>"
  Bus Creator6/1 -> Bus Selector48/1, Bus Selector11/1, Bus Selector9/1
  Bus Selector47/1 -> il0_file3/1  "<signal1>"
  Bus Selector47/2 -> il1_file5/1  "<signal2>"
  Bus Selector47/3 -> il2_file13/1  "<signal3>"
  Bus Selector48/1 -> he0_file7/1  "<He0>"
  Bus Selector48/2 -> he1_file1/1  "<He1>"
  Bus Selector48/3 -> he2_file2/1  "<He2>"
  Bus Creator3/1 -> Bus Selector47/1, Bus Selector26/1, Bus Selector6/1, Bus Selector27/1
  Bus Selector47/4 -> il2_file14/1  "<signal4>"
  Bus Selector47/5 -> il2_file15/1  "<signal5>"
  Bus Selector47/6 -> il0_file9/1  "<signal6>"
  Bus Selector47/7 -> vc1_file2/1  "<signal7>"
  Bus Selector47/8 -> vc2_file2/1  "<signal8>"
  Bus Selector47/9 -> il0_file10/1  "<signal9>"
  Bus Selector47/10 -> il0_file11/1  "<signal10>"
  Bus Selector47/11 -> ilt0_file1/1  "<signal11>"
  Bus Selector47/12 -> ilt1_file2/1  "<signal12>"
  Bus Selector47/13 -> ilt2_file2/1  "<signal13>"
  Bus Selector47/14 -> ilt0_file6/1  "<signal14>"
  Bus Selector47/15 -> ilt0_file2/1  "<signal15>"
  Bus Selector48/4 -> he_file3/1  "<He3>"
  Bus Selector48/5 -> he_file9/1  "<He4>"
  Bus Selector48/6 -> he_file1/1  "<He>"
  Bus Selector48/7 -> he_file2/1  "<H>"
  Bus Selector48/8 -> he0_file9/1  "<H0>"
  Bus Selector48/9 -> he1_file2/1  "<H1>"
  Bus Selector48/10 -> he1_file6/1  "<H2>"
  Bus Selector48/11 -> he0_file8/1  "<H3>"
  Bus Selector48/12 -> he0_file11/1  "<H4>"
  Bus Selector49/1 -> il0_file14/1  "<signal1>"
  Bus Selector49/2 -> il1_file6/1  "<signal2>"
  Bus Selector49/3 -> il2_file16/1  "<signal3>"
  Bus Selector50/1 -> he0_file13/1  "<He0>"
  Bus Selector50/2 -> he1_file7/1  "<He1>"
  Bus Selector50/3 -> he2_file3/1  "<He2>"
  Bus Selector49/4 -> il2_file17/1  "<signal4>"
  Bus Selector49/5 -> il2_file18/1  "<signal5>"
  Bus Selector49/6 -> il0_file15/1  "<signal6>"
  Bus Selector49/7 -> vc1_file3/1  "<signal7>"
  Bus Selector49/8 -> vc2_file3/1  "<signal8>"
  Bus Selector49/9 -> il0_file12/1  "<signal9>"
  Bus Selector49/10 -> il0_file13/1  "<signal10>"
  Bus Selector49/11 -> ilt0_file7/1  "<signal11>"
  Bus Selector49/12 -> ilt1_file3/1  "<signal12>"
  Bus Selector49/13 -> ilt2_file3/1  "<signal13>"
  Bus Selector49/14 -> ilt0_file9/1  "<signal14>"
  Bus Selector49/15 -> ilt0_file8/1  "<signal15>"
  Bus Selector50/4 -> he_file12/1  "<He3>"
  Bus Selector50/5 -> he_file13/1  "<He4>"
  Bus Selector50/6 -> he_file10/1  "<He>"
  Bus Selector50/7 -> he_file11/1  "<H>"
  Bus Selector50/8 -> he0_file15/1  "<H0>"
  Bus Selector50/9 -> he1_file8/1  "<H1>"
  Bus Selector50/10 -> he1_file17/1  "<H2>"
  Bus Selector50/11 -> he0_file14/1  "<H3>"
  Bus Selector50/12 -> he0_file12/1  "<H4>"
  Bus Creator1/1 -> Bus Selector39/1, Bus Selector3/1, Bus Selector49/1, Bus Selector22/1, Bus Selector14/1
